simulink model "Airship_nonlinear_dynamics_simulink"  (R2024b)
settings: Solver=ode15s  StartTime=0.0  StopTime=1000  FixedStep=0.01  MaxStep=0.01  RelTol=1e-5  AbsTol=1e-8
InitFcn:
  | Init
values from neighbouring files (symbols this model uses):
  c = 0.465    [Init.m]    (also in Nonlinear_dynamics.m = 7; init_Skyship.m = 7)
  cf = 0.1395    [Init.m]    (also in Nonlinear_dynamics.m = 3; init_Skyship.m = 3)
  CL_alpha = 5.7    [Init.m]    (also in Nonlinear_dynamics.m; init_Skyship.m)
  D = 1.6    [Init.m]    (also in Nonlinear_dynamics.m = 14; init_Skyship.m = 14)
  delta = deg2rad(10)    [Nonlinear_dynamics.m]    (also in init_Skyship.m = -15)
  delta_e = 0    [Init.m]
  delta_r = 0    [Init.m]
  etaTDF = 1    [Init.m]    (also in Nonlinear_dynamics.m = 0.6; init_Skyship.m = 0.6)
  etaTP = 0.6    [Init.m]    (also in Nonlinear_dynamics.m; init_Skyship.m)
  fProp1 = 0    [Init.m]
  fProp2 = 0    [Init.m]
  fProp_max = 20    [Init.m]
  fTDF = 4000    [Nonlinear_dynamics.m]    (also in init_Skyship.m = 0)
  fTTP = 0    [Init.m]    (also in Nonlinear_dynamics.m = 2000; init_Skyship.m)
  FVN = [5, 5, 5]    [Init.m]    (also in Nonlinear_dynamics.m = 0; init_Skyship.m = 10)
  g = 9.81    [Init.m]    (also in Nonlinear_dynamics.m; init_Skyship.m)
  I33 = eye(3)    [Init.m]    (also in Nonlinear_dynamics.m; init_Skyship.m)
  Ixx = 1.7972    [Init.m]    (also in Nonlinear_dynamics.m = 200658; init_Skyship.m = 200658)
  Ixy = 0    [Init.m]    (also in Nonlinear_dynamics.m; init_Skyship.m)
  Ixz = 0    [Init.m]    (also in Nonlinear_dynamics.m; init_Skyship.m)
  Iyy = 4.9584    [Init.m]    (also in Nonlinear_dynamics.m = 850900; init_Skyship.m = 850900)
  Iyz = 0    [Init.m]    (also in Nonlinear_dynamics.m; init_Skyship.m)
  Izz = 7.9854    [Init.m]    (also in Nonlinear_dynamics.m = 649699; init_Skyship.m = 649699)
  k1 = keta(1)    [Init.m]    (also in Nonlinear_dynamics.m; init_Skyship.m = 0.08; ketaparameters.m = 0)
  k2 = keta(2)    [Init.m]    (also in Nonlinear_dynamics.m; init_Skyship.m = 0.89; ketaparameters.m = 0)
  k_dash = keta(3)    [Init.m]    (also in Nonlinear_dynamics.m; init_Skyship.m = 0.5; ketaparameters.m = 0)
  L = 4.7    [Init.m]    (also in Nonlinear_dynamics.m = zeros(1,4); init_Skyship.m = 52)
  m = 7.31    [Init.m]    (also in Nonlinear_dynamics.m = 5942; init_Skyship.m = 5942; velocity_tf_script.m; velocity_tf_script_v2.m)
  MAF = zeros(6,6)    [Init.m]    (also in Nonlinear_dynamics.m; init_Skyship.m)
  MVN = [0.2, 10, 5]    [Init.m]    (also in Nonlinear_dynamics.m = 0; init_Skyship.m = 0.001)
  p0 = 0    [Init.m]    (also in init_Skyship.m)
  phi0 = 0    [Init.m]    (also in init_Skyship.m)
  Prop1_alpha = 0    [Init.m]
  Prop2_alpha = 0    [Init.m]
  psi0 = 0    [Init.m]    (also in init_Skyship.m)
  q0 = 0    [Init.m]    (also in init_Skyship.m)
  r0 = 0    [Init.m]    (also in init_Skyship.m)
  rGxm = [XG-XB 0 ZG-ZB]'    [Init.m]    (also in Nonlinear_dynamics.m; init_Skyship.m)
  rho_0 = 1.225    [Init.m]    (also in Nonlinear_dynamics.m; init_Skyship.m)
  rho_he = 0.175    [Init.m]
  rTDF1 = [0 0.5 0]'    [Init.m]    (also in Nonlinear_dynamics.m = [3.5 7.87 21]'; init_Skyship.m = [3.5 7.87 21]')
  rTDF2 = [0 -0.5 0]'    [Init.m]    (also in Nonlinear_dynamics.m = [3.5 -7.87 21]'; init_Skyship.m = [3.5 -7.87 21]')
  rTTP = [0 0 0]'    [Init.m]    (also in Nonlinear_dynamics.m = [0 0 20.1]'; init_Skyship.m = [0 0 20.1]')
  Sf = 0.18135    [Init.m]    (also in Nonlinear_dynamics.m = 65; init_Skyship.m = 65)
  t_s = 0.005    [Init.m]
  theta0 = 1    [Init.m]    (also in init_Skyship.m = 0)
  u0 = 0.0    (= 0)    [Init.m]    (also in init_Skyship.m; velocity_tf_script.m = 4; velocity_tf_script_v2.m = 4)
  v0 = 0.0    (= 0)    [Init.m]    (also in init_Skyship.m)
  VB = 5.97    [Init.m]    (also in Nonlinear_dynamics.m = 5153; init_Skyship.m = 4911)
  w0 = 0.0    (= 0)    [Init.m]    (also in init_Skyship.m)
  xE0 = 0    [Init.m]    (also in init_Skyship.m)
  yE0 = 0    [Init.m]    (also in init_Skyship.m)
  zE0 = -h    (= -3.7495)    [Init.m]    (also in init_Skyship.m = -100)
undefined symbols (not defined in the file or in its folder): Sim3dSensor
libraries: slpidlib x13, simulink_extras x4, sim3dcameralib x1, sim3dlib x1, uavsim3dlib x1
(part 2 of 4)

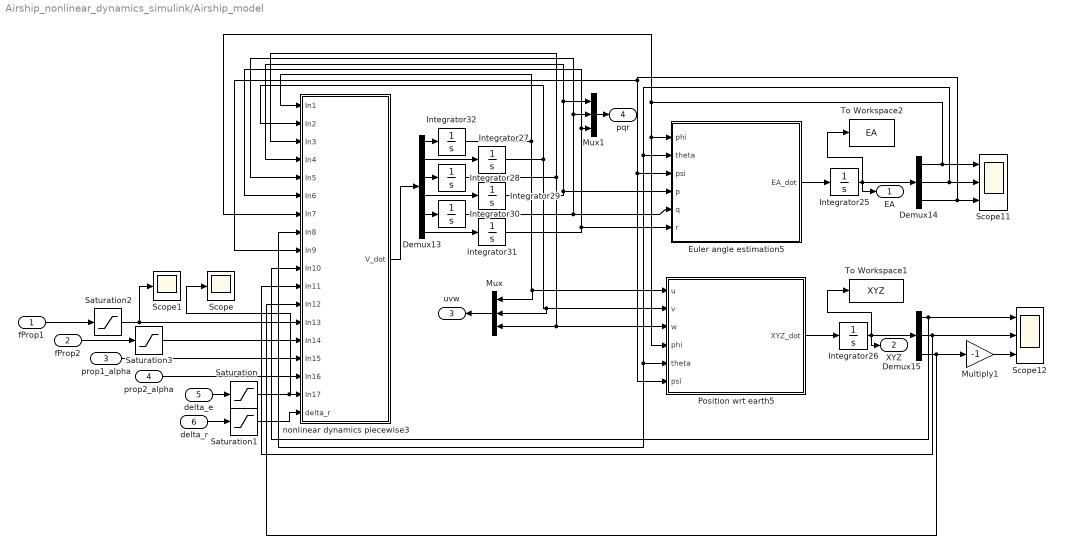
== system Airship_nonlinear_dynamics_simulink/Airship_model ==
  fProp1 : Inport
  fProp2 : Inport  Port=2
  prop1_alpha : Inport  Port=3
  prop2_alpha : Inport  Port=4
  delta_e : Inport  Port=5
  delta_r : Inport  Port=6
  Demux13 : Demux  Outputs=6
  Demux14 : Demux  Outputs=3
  Demux15 : Demux  Outputs=3
  Euler angle estimation5 : MATLAB Function  TreatAsAtomicUnit=on
  Integrator25 : Integrator  InitialCondition=[phi0 theta0 psi0]
  Integrator26 : Integrator  InitialCondition=[xE0 yE0 zE0]
  Integrator27 : Integrator  InitialCondition=v0
  Integrator28 : Integrator  InitialCondition=w0
  Integrator29 : Integrator  InitialCondition=p0
  Integrator30 : Integrator  InitialCondition=q0
  Integrator31 : Integrator  InitialCondition=r0
  Integrator32 : Integrator  InitialCondition=u0
  Multiply1 : Gain  Gain=-1
  Mux : Mux  Inputs=3
  Mux1 : Mux  Inputs=3
  Position wrt earth5 : MATLAB Function  TreatAsAtomicUnit=on
  Saturation : Saturate  UpperLimit=60  LowerLimit=-60
  Saturation1 : Saturate  UpperLimit=60  LowerLimit=-60
  Saturation2 : Saturate  UpperLimit=fProp_max  LowerLimit=-fProp_max
  Saturation3 : Saturate  UpperLimit=fProp_max  LowerLimit=-fProp_max
  Scope : Scope
  Scope1 : Scope
  Scope11 : Scope  NumInputPorts=3
  Scope12 : Scope  NumInputPorts=3
  To Workspace1 : ToWorkspace  VariableName=XYZ  SaveFormat=Timeseries  SampleTime=t_s
  To Workspace2 : ToWorkspace  VariableName=EA  SaveFormat=Timeseries  SampleTime=t_s
  nonlinear dynamics piecewise3 : Subsystem
  EA : Outport
  XYZ : Outport  Port=2
  uvw : Outport  Port=3
  pqr : Outport  Port=4
  wires:
  Demux13/5 -> Integrator30/1
  Integrator27/1 -> nonlinear dynamics piecewise3/2(In2), Position wrt earth5/2(v), Mux/2
  Demux14/2 -> Scope11/2, nonlinear dynamics piecewise3/8(In8), Position wrt earth5/5(theta), Euler angle estimation5/2(theta)
  Demux14/1 -> Scope11/1, nonlinear dynamics piecewise3/7(In7), Position wrt earth5/4(phi), Euler angle estimation5/1(phi)
  Demux13/6 -> Integrator31/1
  Integrator31/1 -> nonlinear dynamics piecewise3/6(In6), Mux1/3, Euler angle estimation5/6(r)
  delta_e/1 -> Saturation/1
  Position wrt earth5/1(XYZ_dot) -> Integrator26/1
  Demux14/3 -> Scope11/3, Euler angle estimation5/3(psi), Position wrt earth5/6(psi), nonlinear dynamics piecewise3/9(In9)
  Integrator28/1 -> nonlinear dynamics piecewise3/3(In3), Position wrt earth5/3(w), Mux/3
  Demux13/4 -> Integrator29/1
  Euler angle estimation5/1(EA_dot) -> Integrator25/1
  Integrator26/1 -> To Workspace1/1, XYZ/1, Demux15/1
  nonlinear dynamics piecewise3/1(V_dot) -> Demux13/1
  Integrator32/1 -> nonlinear dynamics piecewise3/1(In1), Position wrt earth5/1(u), Mux/1
  Demux15/1 -> Scope12/1, nonlinear dynamics piecewise3/10(In10)
  Multiply1/1 -> Scope12/3
  Demux13/1 -> Integrator32/1
  Demux13/2 -> Integrator27/1
  Demux13/3 -> Integrator28/1
  Integrator25/1 -> Demux14/1, EA/1, To Workspace2/1
  Demux15/2 -> nonlinear dynamics piecewise3/11(In11), Scope12/2
  Demux15/3 -> nonlinear dynamics piecewise3/12(In12), Multiply1/1
  fProp1/1 -> Saturation2/1
  prop1_alpha/1 -> nonlinear dynamics piecewise3/15(In15)
  fProp2/1 -> Saturation3/1
  prop2_alpha/1 -> nonlinear dynamics piecewise3/16(In16)
  Mux/1 -> uvw/1
  Integrator29/1 -> Euler angle estimation5/4(p), nonlinear dynamics piecewise3/4(In4), Mux1/1
  Integrator30/1 -> nonlinear dynamics piecewise3/5(In5), Mux1/2, Euler angle estimation5/5(q)
  Mux1/1 -> pqr/1
  delta_r/1 -> Saturation1/1
  Saturation/1 -> Scope/1, nonlinear dynamics piecewise3/17(In17)
  Saturation1/1 -> nonlinear dynamics piecewise3/18(delta_r)
  Saturation2/1 -> Scope1/1, nonlinear dynamics piecewise3/13(In13)
  Saturation3/1 -> nonlinear dynamics piecewise3/14(In14)

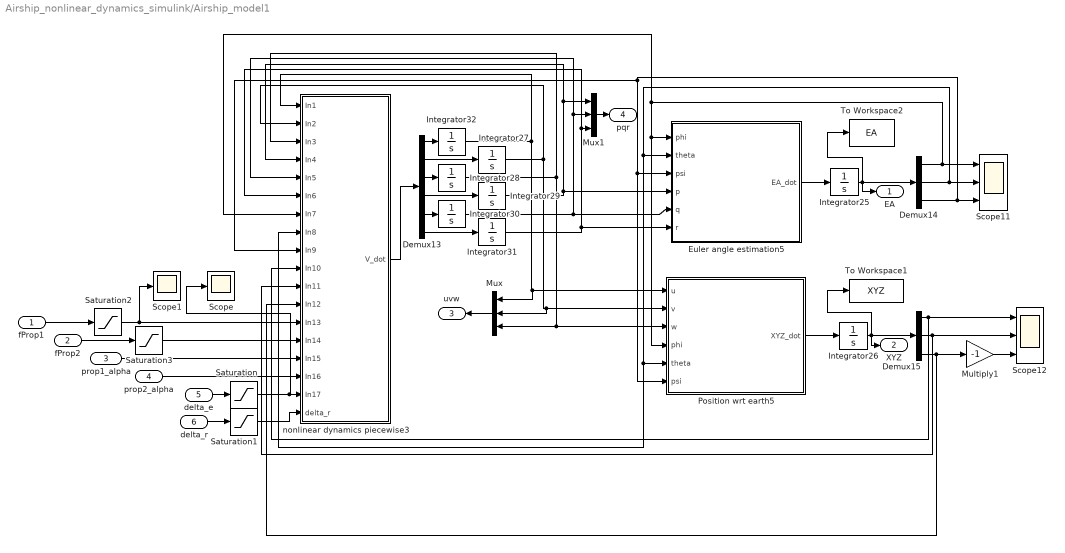
== system Airship_nonlinear_dynamics_simulink/Airship_model1 ==
  fProp1 : Inport
  fProp2 : Inport  Port=2
  prop1_alpha : Inport  Port=3
  prop2_alpha : Inport  Port=4
  delta_e : Inport  Port=5
  delta_r : Inport  Port=6
  Demux13 : Demux  Outputs=6
  Demux14 : Demux  Outputs=3
  Demux15 : Demux  Outputs=3
  Euler angle estimation5 : MATLAB Function  TreatAsAtomicUnit=on
  Integrator25 : Integrator  InitialCondition=[phi0 theta0 psi0]
  Integrator26 : Integrator  InitialCondition=[xE0 yE0 zE0]
  Integrator27 : Integrator  InitialCondition=v0
  Integrator28 : Integrator  InitialCondition=w0
  Integrator29 : Integrator  InitialCondition=p0
  Integrator30 : Integrator  InitialCondition=q0
  Integrator31 : Integrator  InitialCondition=r0
  Integrator32 : Integrator  InitialCondition=u0
  Multiply1 : Gain  Gain=-1
  Mux : Mux  Inputs=3
  Mux1 : Mux  Inputs=3
  Position wrt earth5 : MATLAB Function  TreatAsAtomicUnit=on
  Saturation : Saturate  UpperLimit=60  LowerLimit=-60
  Saturation1 : Saturate  UpperLimit=60  LowerLimit=-60
  Saturation2 : Saturate  UpperLimit=fProp_max  LowerLimit=-fProp_max
  Saturation3 : Saturate  UpperLimit=fProp_max  LowerLimit=-fProp_max
  Scope : Scope
  Scope1 : Scope
  Scope11 : Scope  NumInputPorts=3
  Scope12 : Scope  NumInputPorts=3
  To Workspace1 : ToWorkspace  VariableName=XYZ  SaveFormat=Timeseries  SampleTime=t_s
  To Workspace2 : ToWorkspace  VariableName=EA  SaveFormat=Timeseries  SampleTime=t_s
  nonlinear dynamics piecewise3 : Subsystem
  EA : Outport
  XYZ : Outport  Port=2
  uvw : Outport  Port=3
  pqr : Outport  Port=4
  wires:
  Demux13/5 -> Integrator30/1
  Integrator27/1 -> nonlinear dynamics piecewise3/2(In2), Position wrt earth5/2(v), Mux/2
  Demux14/2 -> Scope11/2, nonlinear dynamics piecewise3/8(In8), Position wrt earth5/5(theta), Euler angle estimation5/2(theta)
  Demux14/1 -> Scope11/1, nonlinear dynamics piecewise3/7(In7), Position wrt earth5/4(phi), Euler angle estimation5/1(phi)
  Demux13/6 -> Integrator31/1
  Integrator31/1 -> nonlinear dynamics piecewise3/6(In6), Mux1/3, Euler angle estimation5/6(r)
  delta_e/1 -> Saturation/1
  Position wrt earth5/1(XYZ_dot) -> Integrator26/1
  Demux14/3 -> Scope11/3, Euler angle estimation5/3(psi), Position wrt earth5/6(psi), nonlinear dynamics piecewise3/9(In9)
  Integrator28/1 -> nonlinear dynamics piecewise3/3(In3), Position wrt earth5/3(w), Mux/3
  Demux13/4 -> Integrator29/1
  Euler angle estimation5/1(EA_dot) -> Integrator25/1
  Integrator26/1 -> To Workspace1/1, XYZ/1, Demux15/1
  nonlinear dynamics piecewise3/1(V_dot) -> Demux13/1
  Integrator32/1 -> nonlinear dynamics piecewise3/1(In1), Position wrt earth5/1(u), Mux/1
  Demux15/1 -> Scope12/1, nonlinear dynamics piecewise3/10(In10)
  Multiply1/1 -> Scope12/3
  Demux13/1 -> Integrator32/1
  Demux13/2 -> Integrator27/1
  Demux13/3 -> Integrator28/1
  Integrator25/1 -> Demux14/1, EA/1, To Workspace2/1
  Demux15/2 -> nonlinear dynamics piecewise3/11(In11), Scope12/2
  Demux15/3 -> nonlinear dynamics piecewise3/12(In12), Multiply1/1
  fProp1/1 -> Saturation2/1
  prop1_alpha/1 -> nonlinear dynamics piecewise3/15(In15)
  fProp2/1 -> Saturation3/1
  prop2_alpha/1 -> nonlinear dynamics piecewise3/16(In16)
  Mux/1 -> uvw/1
  Integrator29/1 -> Euler angle estimation5/4(p), nonlinear dynamics piecewise3/4(In4), Mux1/1
  Integrator30/1 -> nonlinear dynamics piecewise3/5(In5), Mux1/2, Euler angle estimation5/5(q)
  Mux1/1 -> pqr/1
  delta_r/1 -> Saturation1/1
  Saturation/1 -> Scope/1, nonlinear dynamics piecewise3/17(In17)
  Saturation1/1 -> nonlinear dynamics piecewise3/18(delta_r)
  Saturation2/1 -> Scope1/1, nonlinear dynamics piecewise3/13(In13)
  Saturation3/1 -> nonlinear dynamics piecewise3/14(In14)

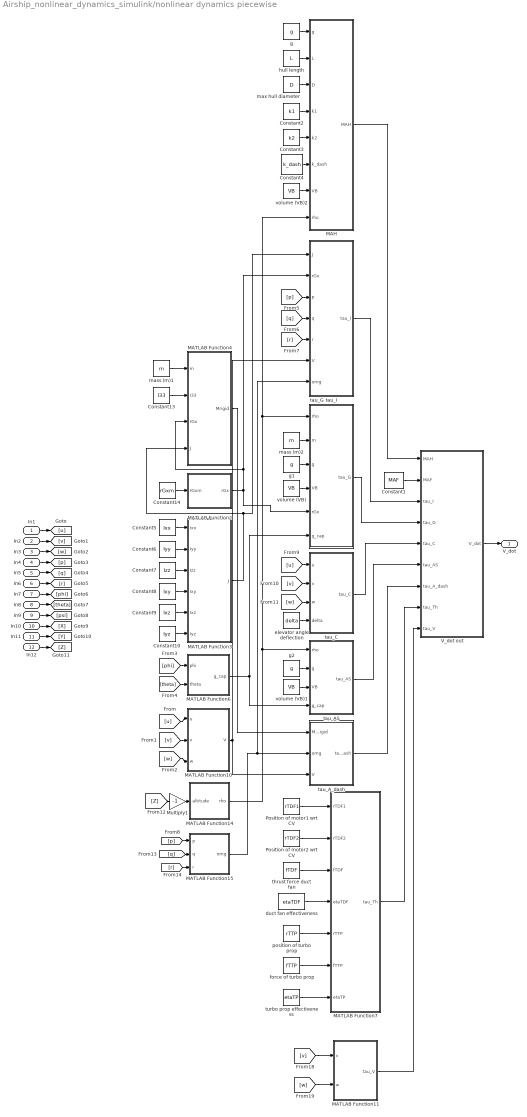
== system Airship_nonlinear_dynamics_simulink/nonlinear dynamics piecewise ==
  In1 : Inport
  In2 : Inport  Port=2
  In3 : Inport  Port=3
  In4 : Inport  Port=4
  In5 : Inport  Port=5
  In6 : Inport  Port=6
  In7 : Inport  Port=7
  In8 : Inport  Port=8
  In9 : Inport  Port=9
  In10 : Inport  Port=10
  In11 : Inport  Port=11
  In12 : Inport  Port=12
  Constant1 : Constant  Value=MAF
  Constant10 : Constant  Value=Iyz
  Constant13 : Constant  Value=I33
  Constant14 : Constant  Value=rGxm
  Constant2 : Constant  Value=k1
  Constant3 : Constant  Value=k2
  Constant4 : Constant  Value=k_dash
  Constant5 : Constant  Value=Ixx
  Constant6 : Constant  Value=Iyy
  Constant7 : Constant  Value=Izz
  Constant8 : Constant  Value=Ixy
  Constant9 : Constant  Value=Ixz
  MAH : MATLAB Function  TreatAsAtomicUnit=on
  MATLAB Function10 : MATLAB Function  TreatAsAtomicUnit=on
  MATLAB Function11 : MATLAB Function  TreatAsAtomicUnit=on
  MATLAB Function14 : MATLAB Function  TreatAsAtomicUnit=on
  MATLAB Function15 : MATLAB Function  TreatAsAtomicUnit=on
  MATLAB Function2 : MATLAB Function  TreatAsAtomicUnit=on
  MATLAB Function3 : MATLAB Function  TreatAsAtomicUnit=on
  MATLAB Function4 : MATLAB Function  TreatAsAtomicUnit=on
  MATLAB Function6 : MATLAB Function  TreatAsAtomicUnit=on
  MATLAB Function7 : MATLAB Function  TreatAsAtomicUnit=on
  Multiply1 : Gain  Gain=-1
  Position of motor1 wrt CV : Constant  Value=rTDF1
  Position of motor2 wrt CV : Constant  Value=rTDF2
  V_dot out : MATLAB Function  TreatAsAtomicUnit=on
  duct fan effectiveness : Constant  Value=etaTDF
  elevator angle deflection : Constant  Value=delta
  force of turbo prop : Constant  Value=fTTP
  g : Constant  Value=g
  g1 : Constant  Value=g
  g2 : Constant  Value=g
  hull length : Constant  Value=L
  mass (m)1 : Constant  Value=m
  mass (m)2 : Constant  Value=m
  max hull diameter : Constant  Value=D
  position of turbo prop : Constant  Value=rTTP
  tau_AS : MATLAB Function  TreatAsAtomicUnit=on
  tau_A_dash : MATLAB Function  TreatAsAtomicUnit=on
  tau_C : MATLAB Function  TreatAsAtomicUnit=on
  tau_G : MATLAB Function  TreatAsAtomicUnit=on
  tau_I : MATLAB Function  TreatAsAtomicUnit=on
  thrust force duct fan : Constant  Value=fTDF
  turbo prop effectiveness : Constant  Value=etaTP
  volume (VB) : Constant  Value=VB
  volume (VB)1 : Constant  Value=VB
  volume (VB)2 : Constant  Value=VB
  V_dot : Outport
  wires:
  V_dot out/1(V_dot) -> V_dot/1
  Constant1/1 -> V_dot out/2(MAF)
  In1/1 -> [u]
  In2/1 -> [v]
  In3/1 -> [w]
  In4/1 -> [p]
  In5/1 -> [q]
  In6/1 -> [r]
  In7/1 -> [phi]
  In8/1 -> [theta]
  In9/1 -> [psi]
  In10/1 -> [X]
  In11/1 -> [Y]
  In12/1 -> [Z]
  mass (m)1/1 -> MATLAB Function4/1(m)
  mass (m)2/1 -> tau_G/2(m)
  Constant13/1 -> MATLAB Function4/2(I33)
  Constant14/1 -> MATLAB Function2/1(rGxm)
  MATLAB Function2/1(rGx) -> tau_G/5(rGx), MATLAB Function4/3(rGx), tau_I/2(rGx)
  MATLAB Function3/1(J) -> MATLAB Function4/4(J), tau_I/1(J)
  Constant6/1 -> MATLAB Function3/2(Iyy)
  Constant5/1 -> MATLAB Function3/1(Ixx)
  Constant7/1 -> MATLAB Function3/3(Izz)
  Constant8/1 -> MATLAB Function3/4(Ixy)
  Constant9/1 -> MATLAB Function3/5(Ixz)
  Constant10/1 -> MATLAB Function3/6(Iyz)
  [u] -> MATLAB Function10/1(u)
  [v] -> MATLAB Function10/2(v)
  [w] -> MATLAB Function10/3(w)
  [phi] -> MATLAB Function6/1(phi)
  [theta] -> MATLAB Function6/2(theta)
  g/1 -> MAH/1(g)
  hull length/1 -> MAH/2(L)
  max hull diameter/1 -> MAH/3(D)
  Constant2/1 -> MAH/4(k1)
  Constant3/1 -> MAH/5(k2)
  [p] -> tau_I/3(p)
  [q] -> tau_I/4(q)
  [r] -> tau_I/5(r)
  MATLAB Function10/1(V) -> tau_A_dash/3(V), tau_I/6(V)
  MATLAB Function14/1(rho) -> tau_AS/1(rho), MAH/8(rho), tau_G/1(rho)
  g1/1 -> tau_G/3(g)
  volume (VB)/1 -> tau_G/4(VB)
  MATLAB Function6/1(g_cap) -> tau_AS/4(g_cap), tau_G/6(g_cap)
  [u] -> tau_C/1(u)
  [v] -> tau_C/2(v)
  [w] -> tau_C/3(w)
  elevator angle deflection/1 -> tau_C/4(delta)
  [Z] -> Multiply1/1
  Multiply1/1 -> MATLAB Function14/1(altitude)
  g2/1 -> tau_AS/2(g)
  volume (VB)1/1 -> tau_AS/3(VB)
  MATLAB Function4/1(Mrigid) -> tau_A_dash/1(MA_rigid)
  [p] -> MATLAB Function15/1(p)
  [q] -> MATLAB Function15/2(q)
  [r] -> MATLAB Function15/3(r)
  MATLAB Function15/1(omg) -> tau_A_dash/2(omg), tau_I/7(omg)
  Position of motor1 wrt CV/1 -> MATLAB Function7/1(rTDF1)
  Position of motor2 wrt CV/1 -> MATLAB Function7/2(rTDF2)
  thrust force duct fan/1 -> MATLAB Function7/3(fTDF)
  duct fan effectiveness/1 -> MATLAB Function7/4(etaTDF)
  position of turbo prop/1 -> MATLAB Function7/5(rTTP)
  force of turbo prop/1 -> MATLAB Function7/6(fTTP)
  turbo prop effectiveness/1 -> MATLAB Function7/7(etaTP)
  [v] -> MATLAB Function11/1(v)
  [w] -> MATLAB Function11/2(w)
  Constant4/1 -> MAH/6(k_dash)
  MAH/1(MAH) -> V_dot out/1(MAH)
  tau_I/1(tau_I) -> V_dot out/3(tau_I)
  tau_G/1(tau_G) -> V_dot out/4(tau_G)
  tau_C/1(tau_C) -> V_dot out/5(tau_C)
  tau_AS/1(tau_AS) -> V_dot out/6(tau_AS)
  tau_A_dash/1(tau_A_dash) -> V_dot out/7(tau_A_dash)
  MATLAB Function7/1(tau_Th) -> V_dot out/8(tau_Th)
  MATLAB Function11/1(tau_V) -> V_dot out/9(tau_V)
  volume (VB)2/1 -> MAH/7(VB)

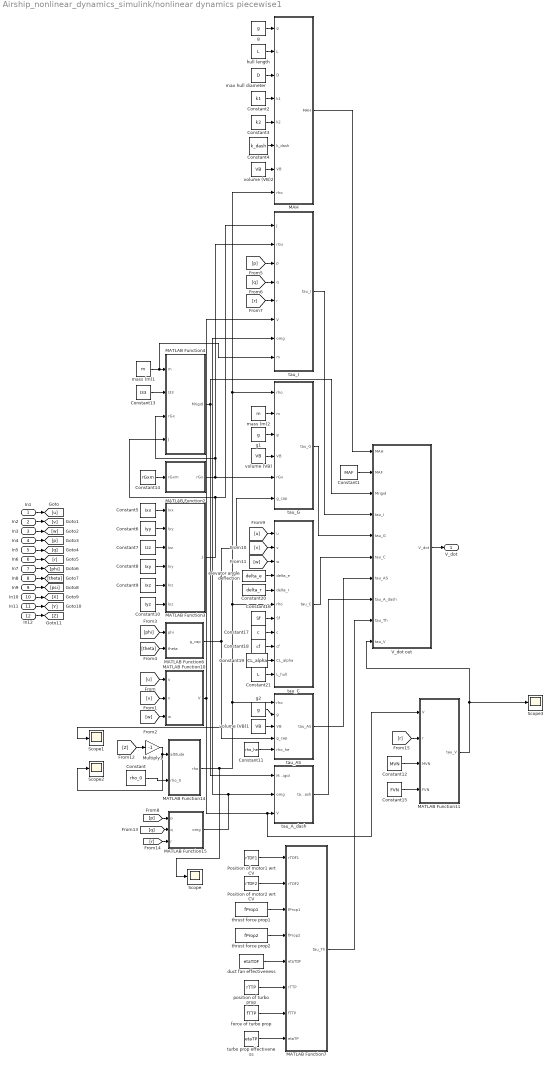
== system Airship_nonlinear_dynamics_simulink/nonlinear dynamics piecewise1 ==
  In1 : Inport
  In2 : Inport  Port=2
  In3 : Inport  Port=3
  In4 : Inport  Port=4
  In5 : Inport  Port=5
  In6 : Inport  Port=6
  In7 : Inport  Port=7
  In8 : Inport  Port=8
  In9 : Inport  Port=9
  In10 : Inport  Port=10
  In11 : Inport  Port=11
  In12 : Inport  Port=12
  Constant : Constant  Value=rho_0
  Constant1 : Constant  Value=MAF
  Constant10 : Constant  Value=Iyz
  Constant11 : Constant  Value=rho_he
  Constant12 : Constant  Value=MVN
  Constant13 : Constant  Value=I33
  Constant14 : Constant  Value=rGxm
  Constant15 : Constant  Value=FVN
  Constant16 : Constant  Value=Sf
  Constant17 : Constant  Value=c
  Constant18 : Constant  Value=cf
  Constant19 : Constant  Value=CL_alpha
  Constant2 : Constant  Value=k1
  Constant20 : Constant  Value=delta_r
  Constant21 : Constant  Value=L
  Constant3 : Constant  Value=k2
  Constant4 : Constant  Value=k_dash
  Constant5 : Constant  Value=Ixx
  Constant6 : Constant  Value=Iyy
  Constant7 : Constant  Value=Izz
  Constant8 : Constant  Value=Ixy
  Constant9 : Constant  Value=Ixz
  MAH : MATLAB Function  TreatAsAtomicUnit=on
  MATLAB Function10 : MATLAB Function  TreatAsAtomicUnit=on
  MATLAB Function11 : MATLAB Function  TreatAsAtomicUnit=on
  MATLAB Function14 : MATLAB Function  TreatAsAtomicUnit=on
  MATLAB Function15 : MATLAB Function  TreatAsAtomicUnit=on
  MATLAB Function2 : MATLAB Function  TreatAsAtomicUnit=on
  MATLAB Function3 : MATLAB Function  TreatAsAtomicUnit=on
  MATLAB Function4 : MATLAB Function  TreatAsAtomicUnit=on
  MATLAB Function6 : MATLAB Function  TreatAsAtomicUnit=on
  MATLAB Function7 : MATLAB Function  TreatAsAtomicUnit=on
  Multiply1 : Gain  Gain=-1
  Position of motor1 wrt CV : Constant  Value=rTDF1
  Position of motor2 wrt CV : Constant  Value=rTDF2
  Scope{,1..3} (4 alike) : Scope
  V_dot out : MATLAB Function  TreatAsAtomicUnit=on
  duct fan effectiveness : Constant  Value=etaTDF
  elevator angle deflection : Constant  Value=delta_e
  force of turbo prop : Constant  Value=fTTP
  g : Constant  Value=g
  g1 : Constant  Value=g
  g2 : Constant  Value=g
  hull length : Constant  Value=L
  mass (m)1 : Constant  Value=m
  mass (m)2 : Constant  Value=m
  max hull diameter : Constant  Value=D
  position of turbo prop : Constant  Value=rTTP
  tau_AS : MATLAB Function  TreatAsAtomicUnit=on
  tau_A_dash : MATLAB Function  TreatAsAtomicUnit=on
  tau_C : MATLAB Function  TreatAsAtomicUnit=on
  tau_G : MATLAB Function  TreatAsAtomicUnit=on
  tau_I : MATLAB Function  TreatAsAtomicUnit=on
  thrust force prop1 : Constant  Value=fProp1
  thrust force prop2 : Constant  Value=fProp2
  turbo prop effectiveness : Constant  Value=etaTP
  volume (VB) : Constant  Value=VB
  volume (VB)1 : Constant  Value=VB
  volume (VB)2 : Constant  Value=VB
  V_dot : Outport
  wires:
  V_dot out/1(V_dot) -> V_dot/1
  Constant1/1 -> V_dot out/2(MAF)
  In1/1 -> [u]
  In2/1 -> [v]
  In3/1 -> [w]
  In4/1 -> [p]
  In5/1 -> [q]
  In6/1 -> [r]
  In7/1 -> [phi]
  In8/1 -> [theta]
  In9/1 -> [psi]
  In10/1 -> [X]
  In11/1 -> [Y]
  In12/1 -> [Z]
  mass (m)1/1 -> tau_I/8(m), MATLAB Function4/1(m)
  mass (m)2/1 -> tau_G/2(m)
  Constant13/1 -> MATLAB Function4/2(I33)
  Constant14/1 -> MATLAB Function2/1(rGxm)
  MATLAB Function2/1(rGx) -> tau_G/5(rGx), MATLAB Function4/3(rGx), tau_I/2(rGx)
  MATLAB Function3/1(J) -> MATLAB Function4/4(J), tau_I/1(J)
  Constant6/1 -> MATLAB Function3/2(Iyy)
  Constant5/1 -> MATLAB Function3/1(Ixx)
  Constant7/1 -> MATLAB Function3/3(Izz)
  Constant8/1 -> MATLAB Function3/4(Ixy)
  Constant9/1 -> MATLAB Function3/5(Ixz)
  Constant10/1 -> MATLAB Function3/6(Iyz)
  [u] -> MATLAB Function10/1(u)
  [v] -> MATLAB Function10/2(v)
  [w] -> MATLAB Function10/3(w)
  [phi] -> MATLAB Function6/1(phi)
  [theta] -> MATLAB Function6/2(theta)
  g/1 -> MAH/1(g)
  hull length/1 -> MAH/2(L)
  max hull diameter/1 -> MAH/3(D)
  Constant2/1 -> MAH/4(k1)
  Constant3/1 -> MAH/5(k2)
  [p] -> tau_I/3(p)
  [q] -> tau_I/4(q)
  [r] -> tau_I/5(r)
  MATLAB Function14/1(rho) -> Scope1/1, MAH/8(rho), tau_G/1(rho), tau_C/6(rho), tau_AS/1(rho), Scope/1
  g1/1 -> tau_G/3(g)
  volume (VB)/1 -> tau_G/4(VB)
  MATLAB Function6/1(g_cap) -> tau_AS/4(g_cap), tau_G/6(g_cap)
  [u] -> tau_C/1(u)
  [v] -> tau_C/2(v)
  [w] -> tau_C/3(w)
  elevator angle deflection/1 -> tau_C/4(delta_e)
  [Z] -> Multiply1/1
  Multiply1/1 -> Scope2/1, MATLAB Function14/1(altitude)
  g2/1 -> tau_AS/2(g)
  volume (VB)1/1 -> tau_AS/3(VB)
  MATLAB Function4/1(Mrigid) -> tau_A_dash/1(MA_rigid), V_dot out/3(Mrigid)
  [p] -> MATLAB Function15/1(p)
  [q] -> MATLAB Function15/2(q)
  [r] -> MATLAB Function15/3(r)
  MATLAB Function15/1(omg) -> tau_I/7(omg), tau_A_dash/2(omg)
  Position of motor1 wrt CV/1 -> MATLAB Function7/1(rTDF1)
  Position of motor2 wrt CV/1 -> MATLAB Function7/2(rTDF2)
  thrust force prop1/1 -> MATLAB Function7/3(fProp1)
  duct fan effectiveness/1 -> MATLAB Function7/5(etaTDF)
  position of turbo prop/1 -> MATLAB Function7/6(rTTP)
  force of turbo prop/1 -> MATLAB Function7/7(fTTP)
  turbo prop effectiveness/1 -> MATLAB Function7/8(etaTP)
  MATLAB Function10/1(V) -> MATLAB Function11/1(V), tau_A_dash/3(V), tau_I/6(V)
  Constant4/1 -> MAH/6(k_dash)
  MAH/1(MAH) -> V_dot out/1(MAH)
  tau_I/1(tau_I) -> V_dot out/4(tau_I)
  tau_G/1(tau_G) -> V_dot out/5(tau_G)
  tau_AS/1(tau_AS) -> V_dot out/7(tau_AS)
  tau_A_dash/1(tau_A_dash) -> V_dot out/8(tau_A_dash)
  MATLAB Function7/1(tau_Th) -> V_dot out/9(tau_Th)
  MATLAB Function11/1(tau_V) -> Scope3/1, V_dot out/10(tau_V)
  volume (VB)2/1 -> MAH/7(VB)
  Constant/1 -> MATLAB Function14/2(rho_0)
  Constant16/1 -> tau_C/7(Sf)
  Constant17/1 -> tau_C/8(c)
  Constant18/1 -> tau_C/9(cf)
  Constant19/1 -> tau_C/10(CL_alpha)
  Constant11/1 -> tau_AS/5(rho_he)
  tau_C/1(tau_C) -> V_dot out/6(tau_C)
  Constant15/1 -> MATLAB Function11/4(FVN)
  Constant12/1 -> MATLAB Function11/3(MVN)
  Constant20/1 -> tau_C/5(delta_r)
  Constant21/1 -> tau_C/11(L_hull)
  [r] -> MATLAB Function11/2(r)
  thrust force prop2/1 -> MATLAB Function7/4(fProp2)

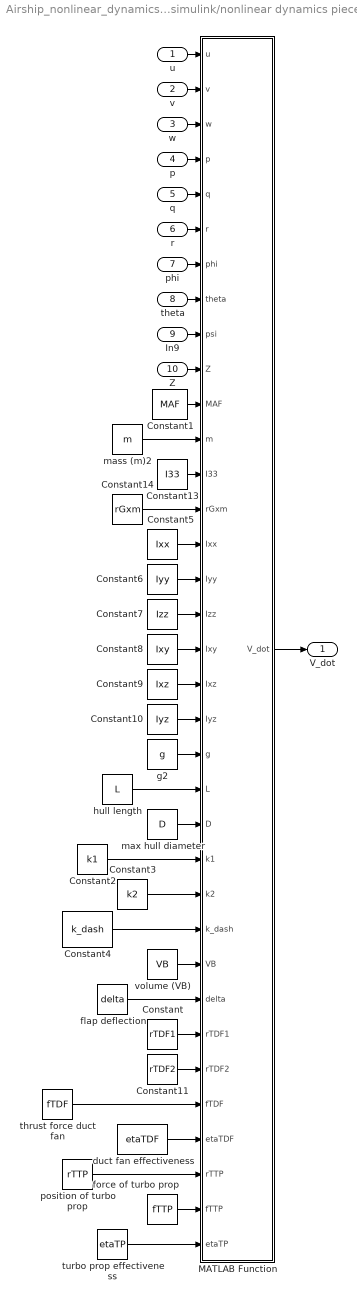
== system Airship_nonlinear_dynamics_simulink/nonlinear dynamics piecewise2 ==
  u : Inport
  v : Inport  Port=2
  w : Inport  Port=3
  p : Inport  Port=4
  q : Inport  Port=5
  r : Inport  Port=6
  phi : Inport  Port=7
  theta : Inport  Port=8
  In9 : Inport  Port=9
  Z : Inport  Port=10
  Constant : Constant  Value=rTDF1
  Constant1 : Constant  Value=MAF
  Constant10 : Constant  Value=Iyz
  Constant11 : Constant  Value=rTDF2
  Constant13 : Constant  Value=I33
  Constant14 : Constant  Value=rGxm
  Constant2 : Constant  Value=k1
  Constant3 : Constant  Value=k2
  Constant4 : Constant  Value=k_dash
  Constant5 : Constant  Value=Ixx
  Constant6 : Constant  Value=Iyy
  Constant7 : Constant  Value=Izz
  Constant8 : Constant  Value=Ixy
  Constant9 : Constant  Value=Ixz
  MATLAB Function : MATLAB Function  TreatAsAtomicUnit=on
  duct fan effectiveness : Constant  Value=etaTDF
  flap deflection : Constant  Value=delta
  force of turbo prop : Constant  Value=fTTP
  g2 : Constant  Value=g
  hull length : Constant  Value=L
  mass (m)2 : Constant  Value=m
  max hull diameter : Constant  Value=D
  position of turbo prop : Constant  Value=rTTP
  thrust force duct fan : Constant  Value=fTDF
  turbo prop effectiveness : Constant  Value=etaTP
  volume (VB) : Constant  Value=VB
  V_dot : Outport
  wires:
  MATLAB Function/1(V_dot) -> V_dot/1
  mass (m)2/1 -> MATLAB Function/12(m)
  Constant6/1 -> MATLAB Function/16(Iyy)
  Constant5/1 -> MATLAB Function/15(Ixx)
  Constant7/1 -> MATLAB Function/17(Izz)
  Constant8/1 -> MATLAB Function/18(Ixy)
  Constant9/1 -> MATLAB Function/19(Ixz)
  Constant10/1 -> MATLAB Function/20(Iyz)
  Constant4/1 -> MATLAB Function/26(k_dash)
  u/1 -> MATLAB Function/1(u)
  v/1 -> MATLAB Function/2(v)
  Constant1/1 -> MATLAB Function/11(MAF)
  Constant13/1 -> MATLAB Function/13(I33)
  g2/1 -> MATLAB Function/21(g)
  Constant14/1 -> MATLAB Function/14(rGxm)
  hull length/1 -> MATLAB Function/22(L)
  max hull diameter/1 -> MATLAB Function/23(D)
  Constant2/1 -> MATLAB Function/24(k1)
  Constant3/1 -> MATLAB Function/25(k2)
  volume (VB)/1 -> MATLAB Function/27(VB)
  flap deflection/1 -> MATLAB Function/28(delta)
  force of turbo prop/1 -> MATLAB Function/34(fTTP)
  position of turbo prop/1 -> MATLAB Function/33(rTTP)
  duct fan effectiveness/1 -> MATLAB Function/32(etaTDF)
  turbo prop effectiveness/1 -> MATLAB Function/35(etaTP)
  thrust force duct fan/1 -> MATLAB Function/31(fTDF)
  Constant/1 -> MATLAB Function/29(rTDF1)
  Constant11/1 -> MATLAB Function/30(rTDF2)
  In9/1 -> MATLAB Function/9(psi)
  w/1 -> MATLAB Function/3(w)
  p/1 -> MATLAB Function/4(p)
  q/1 -> MATLAB Function/5(q)
  r/1 -> MATLAB Function/6(r)
  phi/1 -> MATLAB Function/7(phi)
  theta/1 -> MATLAB Function/8(theta)
  Z/1 -> MATLAB Function/10(Z)

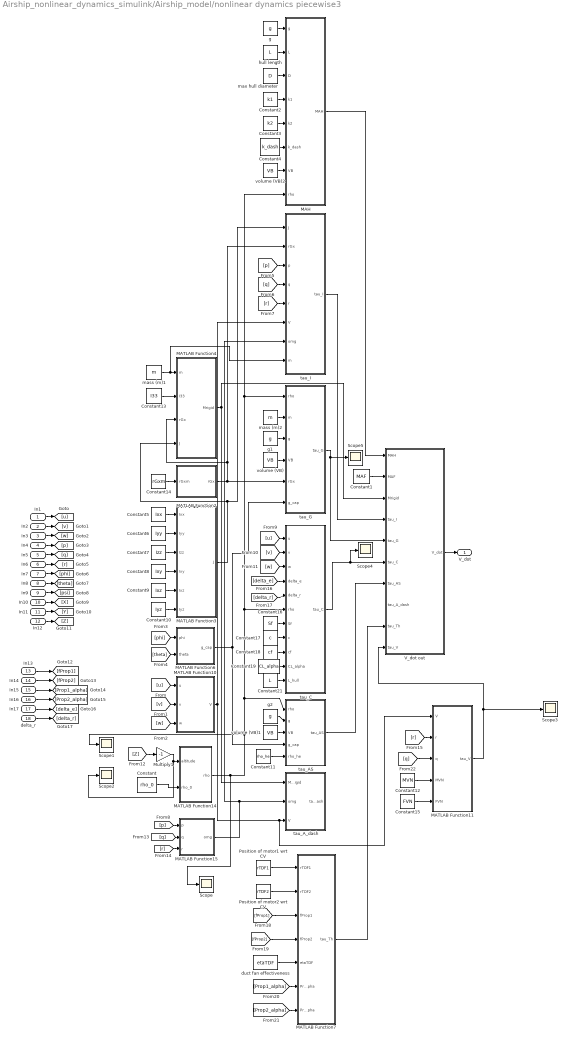
== system Airship_nonlinear_dynamics_simulink/Airship_model/nonlinear dynamics piecewise3 ==
  In1 : Inport
  In2 : Inport  Port=2
  In3 : Inport  Port=3
  In4 : Inport  Port=4
  In5 : Inport  Port=5
  In6 : Inport  Port=6
  In7 : Inport  Port=7
  In8 : Inport  Port=8
  In9 : Inport  Port=9
  In10 : Inport  Port=10
  In11 : Inport  Port=11
  In12 : Inport  Port=12
  In13 : Inport  Port=13
  In14 : Inport  Port=14
  In15 : Inport  Port=15
  In16 : Inport  Port=16
  In17 : Inport  Port=17
  delta_r : Inport  Port=18
  Constant : Constant  Value=rho_0
  Constant1 : Constant  Value=MAF
  Constant10 : Constant  Value=Iyz
  Constant11 : Constant  Value=rho_he
  Constant12 : Constant  Value=MVN
  Constant13 : Constant  Value=I33
  Constant14 : Constant  Value=rGxm
  Constant15 : Constant  Value=FVN
  Constant16 : Constant  Value=Sf
  Constant17 : Constant  Value=c
  Constant18 : Constant  Value=cf
  Constant19 : Constant  Value=CL_alpha
  Constant2 : Constant  Value=k1
  Constant21 : Constant  Value=L
  Constant3 : Constant  Value=k2
  Constant4 : Constant  Value=k_dash
  Constant5 : Constant  Value=Ixx
  Constant6 : Constant  Value=Iyy
  Constant7 : Constant  Value=Izz
  Constant8 : Constant  Value=Ixy
  Constant9 : Constant  Value=Ixz
  MAH : MATLAB Function  TreatAsAtomicUnit=on
  MATLAB Function10 : MATLAB Function  TreatAsAtomicUnit=on
  MATLAB Function11 : MATLAB Function  TreatAsAtomicUnit=on
  MATLAB Function14 : MATLAB Function  TreatAsAtomicUnit=on
  MATLAB Function15 : MATLAB Function  TreatAsAtomicUnit=on
  MATLAB Function2 : MATLAB Function  TreatAsAtomicUnit=on
  MATLAB Function3 : MATLAB Function  TreatAsAtomicUnit=on
  MATLAB Function4 : MATLAB Function  TreatAsAtomicUnit=on
  MATLAB Function6 : MATLAB Function  TreatAsAtomicUnit=on
  MATLAB Function7 : MATLAB Function  TreatAsAtomicUnit=on
  Multiply1 : Gain  Gain=-1
  Position of motor1 wrt CV : Constant  Value=rTDF1
  Position of motor2 wrt CV : Constant  Value=rTDF2
  Scope{,1..5} (6 alike) : Scope
  V_dot out : MATLAB Function  TreatAsAtomicUnit=on
  duct fan effectiveness : Constant  Value=etaTDF
  g : Constant  Value=g
  g1 : Constant  Value=g
  g2 : Constant  Value=g
  hull length : Constant  Value=L
  mass (m)1 : Constant  Value=m
  mass (m)2 : Constant  Value=m
  max hull diameter : Constant  Value=D
  tau_AS : MATLAB Function  TreatAsAtomicUnit=on
  tau_A_dash : MATLAB Function  TreatAsAtomicUnit=on
  tau_C : MATLAB Function  TreatAsAtomicUnit=on
  tau_G : MATLAB Function  TreatAsAtomicUnit=on
  tau_I : MATLAB Function  TreatAsAtomicUnit=on
  volume (VB) : Constant  Value=VB
  volume (VB)1 : Constant  Value=VB
  volume (VB)2 : Constant  Value=VB
  V_dot : Outport
  wires:
  V_dot out/1(V_dot) -> V_dot/1
  Constant1/1 -> V_dot out/2(MAF)
  In1/1 -> [u]
  In2/1 -> [v]
  In3/1 -> [w]
  In4/1 -> [p]
  In5/1 -> [q]
  In6/1 -> [r]
  In7/1 -> [phi]
  In8/1 -> [theta]
  In9/1 -> [psi]
  In10/1 -> [X]
  In11/1 -> [Y]
  In12/1 -> [Z]
  mass (m)1/1 -> tau_I/8(m), MATLAB Function4/1(m)
  mass (m)2/1 -> tau_G/2(m)
  Constant13/1 -> MATLAB Function4/2(I33)
  Constant14/1 -> MATLAB Function2/1(rGxm)
  MATLAB Function2/1(rGx) -> tau_G/5(rGx), MATLAB Function4/3(rGx), tau_I/2(rGx)
  MATLAB Function3/1(J) -> MATLAB Function4/4(J), tau_I/1(J)
  Constant6/1 -> MATLAB Function3/2(Iyy)
  Constant5/1 -> MATLAB Function3/1(Ixx)
  Constant7/1 -> MATLAB Function3/3(Izz)
  Constant8/1 -> MATLAB Function3/4(Ixy)
  Constant9/1 -> MATLAB Function3/5(Ixz)
  Constant10/1 -> MATLAB Function3/6(Iyz)
  [u] -> MATLAB Function10/1(u)
  [v] -> MATLAB Function10/2(v)
  [w] -> MATLAB Function10/3(w)
  [phi] -> MATLAB Function6/1(phi)
  [theta] -> MATLAB Function6/2(theta)
  g/1 -> MAH/1(g)
  hull length/1 -> MAH/2(L)
  max hull diameter/1 -> MAH/3(D)
  Constant2/1 -> MAH/4(k1)
  Constant3/1 -> MAH/5(k2)
  [p] -> tau_I/3(p)
  [q] -> tau_I/4(q)
  [r] -> tau_I/5(r)
  MATLAB Function14/1(rho) -> Scope1/1, MAH/8(rho), tau_G/1(rho), tau_C/6(rho), tau_AS/1(rho), Scope/1
  g1/1 -> tau_G/3(g)
  volume (VB)/1 -> tau_G/4(VB)
  MATLAB Function6/1(g_cap) -> tau_AS/4(g_cap), tau_G/6(g_cap)
  [u] -> tau_C/1(u)
  [v] -> tau_C/2(v)
  [w] -> tau_C/3(w)
  [delta_e] -> tau_C/4(delta_e)
  [Z] -> Multiply1/1
  Multiply1/1 -> Scope2/1, MATLAB Function14/1(altitude)
  g2/1 -> tau_AS/2(g)
  volume (VB)1/1 -> tau_AS/3(VB)
  MATLAB Function4/1(Mrigid) -> tau_A_dash/1(MA_rigid), V_dot out/3(Mrigid)
  [p] -> MATLAB Function15/1(p)
  [q] -> MATLAB Function15/2(q)
  [r] -> MATLAB Function15/3(r)
  MATLAB Function15/1(omg) -> tau_I/7(omg), tau_A_dash/2(omg)
  Position of motor1 wrt CV/1 -> MATLAB Function7/1(rTDF1)
  Position of motor2 wrt CV/1 -> MATLAB Function7/2(rTDF2)
  duct fan effectiveness/1 -> MATLAB Function7/5(etaTDF)
  [fProp1] -> MATLAB Function7/3(fProp1)
  MATLAB Function10/1(V) -> MATLAB Function11/1(V), tau_A_dash/3(V), tau_I/6(V)
  Constant4/1 -> MAH/6(k_dash)
  MAH/1(MAH) -> V_dot out/1(MAH)
  tau_I/1(tau_I) -> V_dot out/4(tau_I)
  tau_G/1(tau_G) -> Scope5/1, V_dot out/5(tau_G)
  tau_AS/1(tau_AS) -> V_dot out/7(tau_AS)
  MATLAB Function11/1(tau_V) -> V_dot out/10(tau_V), Scope3/1
  volume (VB)2/1 -> MAH/7(VB)
  Constant/1 -> MATLAB Function14/2(rho_0)
  Constant16/1 -> tau_C/7(Sf)
  Constant17/1 -> tau_C/8(c)
  Constant18/1 -> tau_C/9(cf)
  Constant19/1 -> tau_C/10(CL_alpha)
  Constant11/1 -> tau_AS/5(rho_he)
  tau_C/1(tau_C) -> Scope4/1, V_dot out/6(tau_C)
  Constant15/1 -> MATLAB Function11/5(FVN)
  Constant12/1 -> MATLAB Function11/4(MVN)
  [delta_r] -> tau_C/5(delta_r)
  Constant21/1 -> tau_C/11(L_hull)
  [r] -> MATLAB Function11/2(r)
  In13/1 -> [fProp1]
  In14/1 -> [fProp2]
  In15/1 -> [Prop1_alpha]
  In16/1 -> [Prop2_alpha]
  In17/1 -> [delta_e]
  delta_r/1 -> [delta_r]
  [fProp2] -> MATLAB Function7/4(fProp2)
  [Prop1_alpha] -> MATLAB Function7/6(Prop1_alpha)
  [Prop2_alpha] -> MATLAB Function7/7(Prop2_alpha)
  [q] -> MATLAB Function11/3(q)
  MATLAB Function7/1(tau_Th) -> V_dot out/9(tau_Th)

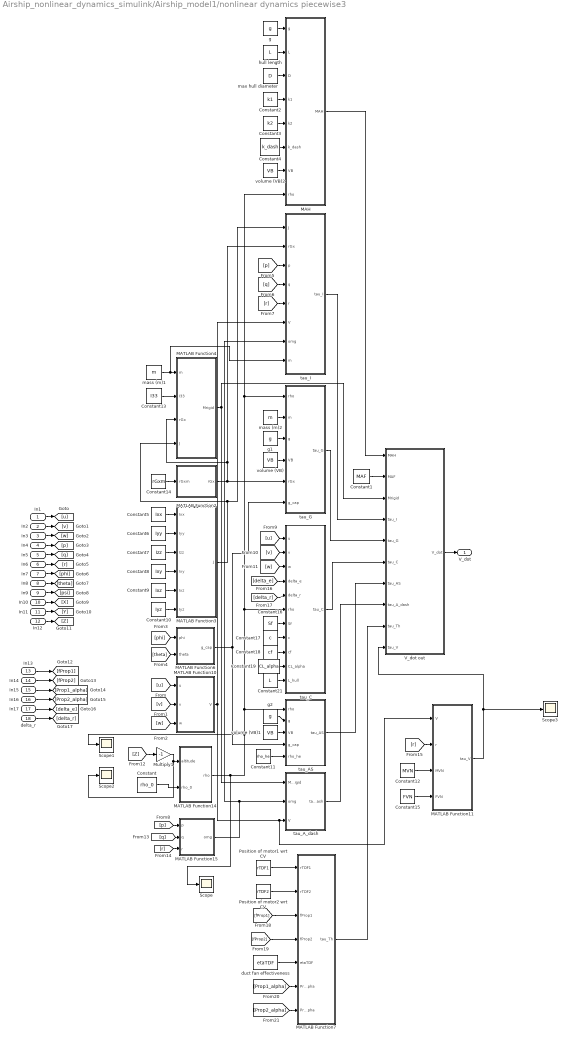
== system Airship_nonlinear_dynamics_simulink/Airship_model1/nonlinear dynamics piecewise3 ==
  In1 : Inport
  In2 : Inport  Port=2
  In3 : Inport  Port=3
  In4 : Inport  Port=4
  In5 : Inport  Port=5
  In6 : Inport  Port=6
  In7 : Inport  Port=7
  In8 : Inport  Port=8
  In9 : Inport  Port=9
  In10 : Inport  Port=10
  In11 : Inport  Port=11
  In12 : Inport  Port=12
  In13 : Inport  Port=13
  In14 : Inport  Port=14
  In15 : Inport  Port=15
  In16 : Inport  Port=16
  In17 : Inport  Port=17
  delta_r : Inport  Port=18
  Constant : Constant  Value=rho_0
  Constant1 : Constant  Value=MAF
  Constant10 : Constant  Value=Iyz
  Constant11 : Constant  Value=rho_he
  Constant12 : Constant  Value=MVN
  Constant13 : Constant  Value=I33
  Constant14 : Constant  Value=rGxm
  Constant15 : Constant  Value=FVN
  Constant16 : Constant  Value=Sf
  Constant17 : Constant  Value=c
  Constant18 : Constant  Value=cf
  Constant19 : Constant  Value=CL_alpha
  Constant2 : Constant  Value=k1
  Constant21 : Constant  Value=L
  Constant3 : Constant  Value=k2
  Constant4 : Constant  Value=k_dash
  Constant5 : Constant  Value=Ixx
  Constant6 : Constant  Value=Iyy
  Constant7 : Constant  Value=Izz
  Constant8 : Constant  Value=Ixy
  Constant9 : Constant  Value=Ixz
  MAH : MATLAB Function  TreatAsAtomicUnit=on
  MATLAB Function10 : MATLAB Function  TreatAsAtomicUnit=on
  MATLAB Function11 : MATLAB Function  TreatAsAtomicUnit=on
  MATLAB Function14 : MATLAB Function  TreatAsAtomicUnit=on
  MATLAB Function15 : MATLAB Function  TreatAsAtomicUnit=on
  MATLAB Function2 : MATLAB Function  TreatAsAtomicUnit=on
  MATLAB Function3 : MATLAB Function  TreatAsAtomicUnit=on
  MATLAB Function4 : MATLAB Function  TreatAsAtomicUnit=on
  MATLAB Function6 : MATLAB Function  TreatAsAtomicUnit=on
  MATLAB Function7 : MATLAB Function  TreatAsAtomicUnit=on
  Multiply1 : Gain  Gain=-1
  Position of motor1 wrt CV : Constant  Value=rTDF1
  Position of motor2 wrt CV : Constant  Value=rTDF2
  Scope{,1..3} (4 alike) : Scope
  V_dot out : MATLAB Function  TreatAsAtomicUnit=on
  duct fan effectiveness : Constant  Value=etaTDF
  g : Constant  Value=g
  g1 : Constant  Value=g
  g2 : Constant  Value=g
  hull length : Constant  Value=L
  mass (m)1 : Constant  Value=m
  mass (m)2 : Constant  Value=m
  max hull diameter : Constant  Value=D
  tau_AS : MATLAB Function  TreatAsAtomicUnit=on
  tau_A_dash : MATLAB Function  TreatAsAtomicUnit=on
  tau_C : MATLAB Function  TreatAsAtomicUnit=on
  tau_G : MATLAB Function  TreatAsAtomicUnit=on
  tau_I : MATLAB Function  TreatAsAtomicUnit=on
  volume (VB) : Constant  Value=VB
  volume (VB)1 : Constant  Value=VB
  volume (VB)2 : Constant  Value=VB
  V_dot : Outport
  wires:
  V_dot out/1(V_dot) -> V_dot/1
  Constant1/1 -> V_dot out/2(MAF)
  In1/1 -> [u]
  In2/1 -> [v]
  In3/1 -> [w]
  In4/1 -> [p]
  In5/1 -> [q]
  In6/1 -> [r]
  In7/1 -> [phi]
  In8/1 -> [theta]
  In9/1 -> [psi]
  In10/1 -> [X]
  In11/1 -> [Y]
  In12/1 -> [Z]
  mass (m)1/1 -> tau_I/8(m), MATLAB Function4/1(m)
  mass (m)2/1 -> tau_G/2(m)
  Constant13/1 -> MATLAB Function4/2(I33)
  Constant14/1 -> MATLAB Function2/1(rGxm)
  MATLAB Function2/1(rGx) -> tau_G/5(rGx), MATLAB Function4/3(rGx), tau_I/2(rGx)
  MATLAB Function3/1(J) -> MATLAB Function4/4(J), tau_I/1(J)
  Constant6/1 -> MATLAB Function3/2(Iyy)
  Constant5/1 -> MATLAB Function3/1(Ixx)
  Constant7/1 -> MATLAB Function3/3(Izz)
  Constant8/1 -> MATLAB Function3/4(Ixy)
  Constant9/1 -> MATLAB Function3/5(Ixz)
  Constant10/1 -> MATLAB Function3/6(Iyz)
  [u] -> MATLAB Function10/1(u)
  [v] -> MATLAB Function10/2(v)
  [w] -> MATLAB Function10/3(w)
  [phi] -> MATLAB Function6/1(phi)
  [theta] -> MATLAB Function6/2(theta)
  g/1 -> MAH/1(g)
  hull length/1 -> MAH/2(L)
  max hull diameter/1 -> MAH/3(D)
  Constant2/1 -> MAH/4(k1)
  Constant3/1 -> MAH/5(k2)
  [p] -> tau_I/3(p)
  [q] -> tau_I/4(q)
  [r] -> tau_I/5(r)
  MATLAB Function14/1(rho) -> Scope1/1, MAH/8(rho), tau_G/1(rho), tau_C/6(rho), tau_AS/1(rho), Scope/1
  g1/1 -> tau_G/3(g)
  volume (VB)/1 -> tau_G/4(VB)
  MATLAB Function6/1(g_cap) -> tau_AS/4(g_cap), tau_G/6(g_cap)
  [u] -> tau_C/1(u)
  [v] -> tau_C/2(v)
  [w] -> tau_C/3(w)
  [delta_e] -> tau_C/4(delta_e)
  [Z] -> Multiply1/1
  Multiply1/1 -> Scope2/1, MATLAB Function14/1(altitude)
  g2/1 -> tau_AS/2(g)
  volume (VB)1/1 -> tau_AS/3(VB)
  MATLAB Function4/1(Mrigid) -> tau_A_dash/1(MA_rigid), V_dot out/3(Mrigid)
  [p] -> MATLAB Function15/1(p)
  [q] -> MATLAB Function15/2(q)
  [r] -> MATLAB Function15/3(r)
  MATLAB Function15/1(omg) -> tau_I/7(omg), tau_A_dash/2(omg)
  Position of motor1 wrt CV/1 -> MATLAB Function7/1(rTDF1)
  Position of motor2 wrt CV/1 -> MATLAB Function7/2(rTDF2)
  duct fan effectiveness/1 -> MATLAB Function7/5(etaTDF)
  [fProp1] -> MATLAB Function7/3(fProp1)
  MATLAB Function10/1(V) -> MATLAB Function11/1(V), tau_A_dash/3(V), tau_I/6(V)
  Constant4/1 -> MAH/6(k_dash)
  MAH/1(MAH) -> V_dot out/1(MAH)
  tau_I/1(tau_I) -> V_dot out/4(tau_I)
  tau_G/1(tau_G) -> V_dot out/5(tau_G)
  tau_AS/1(tau_AS) -> V_dot out/7(tau_AS)
  tau_A_dash/1(tau_A_dash) -> V_dot out/8(tau_A_dash)
  MATLAB Function7/1(tau_Th) -> V_dot out/9(tau_Th)
  MATLAB Function11/1(tau_V) -> Scope3/1, V_dot out/10(tau_V)
  volume (VB)2/1 -> MAH/7(VB)
  Constant/1 -> MATLAB Function14/2(rho_0)
  Constant16/1 -> tau_C/7(Sf)
  Constant17/1 -> tau_C/8(c)
  Constant18/1 -> tau_C/9(cf)
  Constant19/1 -> tau_C/10(CL_alpha)
  Constant11/1 -> tau_AS/5(rho_he)
  tau_C/1(tau_C) -> V_dot out/6(tau_C)
  Constant15/1 -> MATLAB Function11/4(FVN)
  Constant12/1 -> MATLAB Function11/3(MVN)
  [delta_r] -> tau_C/5(delta_r)
  Constant21/1 -> tau_C/11(L_hull)
  [r] -> MATLAB Function11/2(r)
  In13/1 -> [fProp1]
  In14/1 -> [fProp2]
  In15/1 -> [Prop1_alpha]
  In16/1 -> [Prop2_alpha]
  In17/1 -> [delta_e]
  delta_r/1 -> [delta_r]
  [fProp2] -> MATLAB Function7/4(fProp2)
  [Prop1_alpha] -> MATLAB Function7/6(Prop1_alpha)
  [Prop2_alpha] -> MATLAB Function7/7(Prop2_alpha)

== matlab function Airship_nonlinear_dynamics_simulink/Position wrt earth1 ==
  data: u input; XYZ_dot output; v input; w input; phi input; theta input; psi input
function XYZ_dot = position_wrt_Earth(u,v,w,phi,theta,psi)


R_be = [cos(theta)*cos(psi) , sin(theta)*sin(phi)*cos(psi) - cos(theta)*sin(psi), cos(phi)*cos(psi)*sin(theta)+ sin(phi)*sin(psi); ...
    cos(theta)*sin(psi), sin(phi)*sin(theta)*sin(psi) + cos(phi)*cos(psi), cos(phi)*sin(theta)*sin(psi) - sin(phi)*cos(psi); ...
    -sin(theta) , sin(phi)*cos(theta) , cos(phi)*cos(theta)];

body_velocity = [u; v; w];
XYZ_dot = transpose(R_be*body_velocity);
end

== matlab function Airship_nonlinear_dynamics_simulink/nonlinear dynamics piecewise/tau_G ==
  data: rho input; tau_G output size=[6, 1]; m input; g input; VB input; rGx input; g_cap input
function tau_G = fcn(rho, m, g, VB, rGx, g_cap)
%% Gravitational forces and moments


w = m*g;
B = VB*rho*g;
FG = w*g_cap; % Weight component in body frame (N)
tau_G = [FG; rGx*FG];

== matlab function Airship_nonlinear_dynamics_simulink/nonlinear dynamics piecewise/MATLAB Function2 ==
  data: rGxm input; rGx output
function rGx = fcn(rGxm)
rGx = [0 -rGxm(3) rGxm(2) ; rGxm(3) 0 -rGxm(1) ; -rGxm(2) rGxm(1) 0];

== matlab function Airship_nonlinear_dynamics_simulink/nonlinear dynamics piecewise/MATLAB Function3 ==
  data: Ixx input; J output; Iyy input; Izz input; Ixy input; Ixz input; Iyz input
function J = fcn(Ixx, Iyy, Izz, Ixy, Ixz, Iyz)
J = [ Ixx, Ixy, Ixz ; Ixy, Iyy, Iyz ; Ixz, Iyz, Izz];

== matlab function Airship_nonlinear_dynamics_simulink/nonlinear dynamics piecewise/MATLAB Function4 ==
  data: m input; Mrigid output; I33 input; rGx input; J input
function Mrigid = fcn(m, I33, rGx, J)
Mrigid = [m*I33, -m*rGx; m*rGx,  J];

== matlab function Airship_nonlinear_dynamics_simulink/nonlinear dynamics piecewise/tau_AS ==
  data: rho input; tau_AS output size=[6, 1]; g input; VB input; g_cap input
function tau_AS = fcn(rho, g, VB, g_cap)
%% Aerostatic forces and moments

% first three are forces along x y z
% next three are moments along x y z 
rv = [0 0 0]'; %Since body frame is established at CV, the position ...
FAS = -rho*g*VB*g_cap; %Aerostatic forces N
tau_AS = [FAS; cross(rv,FAS)]; %Aerostatic forces and moments

== matlab function Airship_nonlinear_dynamics_simulink/nonlinear dynamics piecewise/MATLAB Function6 ==
  data: phi input; g_cap output; theta input
function g_cap = fcn(phi, theta)
g_cap = [-sin(theta), cos(theta)*sin(phi), cos(theta)*cos(phi)]';

== matlab function Airship_nonlinear_dynamics_simulink/nonlinear dynamics piecewise/MATLAB Function7 ==
  data: rTDF1 input; tau_Th output; rTDF2 input; fTDF input; etaTDF input; rTTP input; fTTP input; etaTP input
function tau_Th = fcn(rTDF1, rTDF2, fTDF, etaTDF, rTTP,  fTTP,  etaTP)
%% Airship thrust force and moments


FTDF1 = etaTDF * [fTDF 0 0 ]'; %Thrust force N
FTDF2 = etaTDF * [fTDF 0 0 ]';
FTDF = FTDF1+FTDF2;
MTDF1 = cross(rTDF1, FTDF1); %Moments N-m
MTDF2 = cross(rTDF2, FTDF2);
MTDF = MTDF1 + MTDF2;


FTTP = etaTP* [fTTP 0 0 ]';
MTTP = cross(rTTP, FTTP);

FT = FTTP + FTDF;
MT = MTTP + MTDF;
tau_Th = [FT; MT];

== matlab function Airship_nonlinear_dynamics_simulink/nonlinear dynamics piecewise/MAH ==
  data: MAH output; g input; L input; D input; k1 input; k2 input; k_dash input; VB input; rho input
function MAH = fcn(g, L, D, k1, k2, k_dash, VB, rho)
%% Estimation of added mass matrix
% MAH - added mass of airship hull
B = VB*rho*g; %Bouyancy force
m_dash = B/g;
%I_dash = sum(m_dash * (L.^2 + D^2) / 20); 
I_dash = (m_dash * (L.^2 + D^2) / 20); 

mH11 = k1*m_dash;
mH22 = k2*m_dash;
mH33 = mH22;
mH44 = 0;
mH55 = k_dash*I_dash;
mH66 = mH55;
mH = [mH11, mH22, mH33, mH44, mH55, mH66];

MAH = diag(mH); %6x6 diagonal matrix

== matlab function Airship_nonlinear_dynamics_simulink/nonlinear dynamics piecewise/tau_A_dash ==
  data: MA_rigid input; tau_A_dash output size=[6, 1]; omg input; V input
function tau_A_dash = fcn(MA_rigid, omg, V)
%% Aerodynamic forces and moments
% symmetric added mass axis
% Aerodynamic forces N and moments N-m

%extract components from the syymetric added mass axis
M11 = MA_rigid(1:3, 1:3);
M12 = MA_rigid(1:3, 4:6);
M21 = MA_rigid(4:6, 1:3);
M22 = MA_rigid(4:6, 4:6);

% Calc aero forces and moments

forces_due_to_rotation = cross(omg, (M11 * V + M12 *omg));
moments_due_to_translation = cross(V, (M11*V+M12*omg));
moments_due_to_rotation = cross (omg, (M21*V + M22*omg));

tau_A_dash = zeros(6,1);
%combine into aero forces and moments (sign change - to +)
tau_A_dash = [forces_due_to_rotation; moments_due_to_translation+moments_due_to_rotation];

== matlab function Airship_nonlinear_dynamics_simulink/nonlinear dynamics piecewise/MATLAB Function10 ==
  data: u input; V output; v input; w input
function V = fcn(u, v, w)
V = [u v w]';

== matlab function Airship_nonlinear_dynamics_simulink/nonlinear dynamics piecewise/MATLAB Function11 ==
  data: v input; tau_V output; w input
function tau_V = fcn(v, w)
%% Viscous forces
FVN = 0; %Viscous force
MVN = 0; %Viscous Moment
FV = FVN*[0 (-v/sqrt(v^2 + w^2)) (-w/sqrt(v^2 +w^2)) ]';
MV = MVN*[0 (w/sqrt(v^2 + w^2)) (-v/sqrt(v^2 +w^2)) ]';
tau_V = [FV; MV];

%tau_V = [0 0 0 0 0 0]'; %if slow speed

== matlab function Airship_nonlinear_dynamics_simulink/nonlinear dynamics piecewise/V_dot out ==
  data: MAH input; V_dot output; MAF input; tau_I input; tau_G input; tau_C input; tau_AS input; tau_A_dash input; tau_Th input; tau_V input
function V_dot = fcn(MAH, MAF, tau_I, tau_G, tau_C, tau_AS, tau_A_dash, tau_Th, tau_V)
%% Return
V_dot = zeros(6,1);
MA_rigid = (MAH+MAF);


%                                       +tau_Imp for gusts
V_dot = (MA_rigid + Mrigid) \ (tau_I + tau_G + tau_C + tau_AS + tau_A_dash + tau_Th + tau_V);

== matlab function Airship_nonlinear_dynamics_simulink/nonlinear dynamics piecewise/tau_C ==
  data: u input; tau_C output size=[6, 1]; v input; w input; delta input
function tau_C = fcn(u, v, w, delta)
%% Control forces and moments
% Constants

 V_bar  = sqrt(v^2 + u^2 + w^2) ; %true airspeed in m/s
 Sf = 65; % Surface area of the fin m^2
 c= 7 ; % Chord length of the fin
 cf = 3; %Flap chord
 
 S_FE = 65; %reference surface area m^2
 %
 delta = deg2rad(10);
 %lift curve slope
 CL_alpha = 5.7; %Change as needed
 
 %theoretical effectiveness factor tau
 theta_f = acos(2*cf/c -1);
 tau = 1- (theta_f - sin(theta_f)) /pi;
 
 %correction factor eta_d
 eta_d = 0.8; %simplified fucntion
 %3D effectiveness value
 k3D = 1.2; %example value
 %calc DeltaCL
 
 DeltaCL = CL_alpha *tau * eta_d * k3D * delta;
 
 DeltaCD = 1.7* (cf/c)^1.38 * (Sf / S_FE) * sin(delta)^2;
 
 %Moment calcs for each fin
 numerator = -2*sin(theta_f) - sin(2*theta_f);
 denominator = 8 * (pi - theta_f + sin(theta_f));
 
 ratio = numerator/denominator;
 
 DeltaCM1_4 = ratio*DeltaCL;
 
 %Deflection anges degrees
 theta = [45, 135, 225, 315];
 
 %initialize force and moment arrays
 
 Fx = zeros(1,4);
 Fy = zeros(1,4);
 Fz = zeros(1,4);
 
 L = zeros(1,4);
 M = zeros(1,4);
 N = zeros(1,4);
 
 %calc forces and moements for each fin
 
 for i = 1:4
     %conv theta to radians
     theta_rad = deg2rad(theta(i));
 
     %calc forces
     Fx(i) = -0.5 * rho * V_bar^2 *Sf*DeltaCD;
     Fy(i) = 0.5*rho*V_bar^2*Sf*(DeltaCL *sin(theta_rad)+ DeltaCD * cos(theta_rad));
     Fz(i) = -0.5 * rho * V_bar^2 *Sf*(DeltaCL *cos(theta_rad)- DeltaCD * sin(theta_rad));
 
     L(i) = Fz(i); %Assume y_i = 1 for simplicity
     M(i) = 0.5*rho*V_bar^2*Sf*c*DeltaCM1_4;
     N(i) = Fy(i); %Assume x_i = 1 for simplicity 
 end
 % Totals
 TotalFx = sum(Fx(:));
 TotalFy = sum(Fy(:));
 TotalFz = sum(Fz(:));
 
 TotalL = sum(L(:));
 TotalM = sum(M(:));
 TotalN = sum(N(:));

 tau_C = [TotalFx TotalFy TotalFz TotalL TotalM TotalN]';

%For natural response 
tau_C = [0 0 0 0 0 0]';

== matlab function Airship_nonlinear_dynamics_simulink/nonlinear dynamics piecewise/MATLAB Function14 ==
  data: altitude input; rho output
function rho = fcn(altitude)
%Atmosphere model
rho_0 = 1.225; %Density at sea level in kg/m3
H = 8400; %Scale height in meters;

%alitude range
%altitude = -airship(12); %linspace(0,12000, 500); %Altitude from 0 to 12000 m

density = rho_0 *exp(-altitude / H );
rho = density;

== matlab function Airship_nonlinear_dynamics_simulink/nonlinear dynamics piecewise/MATLAB Function15 ==
  data: p input; omg output; q input; r input
function omg = fcn(p, q, r)
omg = [p q r]';

== matlab function Airship_nonlinear_dynamics_simulink/Euler angle estimation3 ==
  data: phi input; EA_dot output; theta input; psi input; p input; q input; r input
function EA_dot = Euler_angle_estimation(phi, theta, psi,p, q, r)


E_dot = [1, sin(phi)* tan(theta) , cos(phi)*tan(theta);
         0, cos(phi) , -sin(phi);
         0, sin(phi)/cos(theta), cos(phi)/cos(theta)];

body_rates = [p; q; r];

EA_dot = transpose(E_dot*body_rates);

end

== matlab function Airship_nonlinear_dynamics_simulink/Position wrt earth3 ==
  data: u input; XYZ_dot output; v input; w input; phi input; theta input; psi input
function XYZ_dot = position_wrt_Earth(u,v,w,phi,theta,psi)


R_be = [cos(theta)*cos(psi) , sin(theta)*sin(phi)*cos(psi) - cos(theta)*sin(psi), cos(phi)*cos(psi)*sin(theta)+ sin(phi)*sin(psi); ...
    cos(theta)*sin(psi), sin(phi)*sin(theta)*sin(psi) + cos(phi)*cos(psi), cos(phi)*sin(theta)*sin(psi) - sin(phi)*cos(psi); ...
    -sin(theta) , sin(phi)*cos(theta) , cos(phi)*cos(theta)];

body_velocity = [u; v; w];
XYZ_dot = transpose(R_be*body_velocity);
end

== matlab function Airship_nonlinear_dynamics_simulink/nonlinear dynamics piecewise1/MAH ==
  data: MAH output; g input; L input; D input; k1 input; k2 input; k_dash input; VB input; rho input
function MAH = fcn(g, L, D, k1, k2, k_dash, VB, rho)
%% Estimation of added mass matrix
% MAH - added mass of airship hull
B = VB*rho*g; %Bouyancy force
m_dash = B/g;
%I_dash = sum(m_dash * (L.^2 + D^2) / 20); 
I_dash = (m_dash * (L.^2 + D^2) / 20); 

mH11 = k1*m_dash;
mH22 = k2*m_dash;
mH33 = mH22;
mH44 = 0;
mH55 = k_dash*I_dash;
mH66 = mH55;
mH = [mH11, mH22, mH33, mH44, mH55, mH66];

MAH = diag(mH); %6x6 diagonal matrix
end

== matlab function Airship_nonlinear_dynamics_simulink/nonlinear dynamics piecewise1/MATLAB Function10 ==
  data: u input; V output; v input; w input
function V = fcn(u, v, w)
V = [u v w]';
end

== matlab function Airship_nonlinear_dynamics_simulink/nonlinear dynamics piecewise1/MATLAB Function11 ==
  data: V input; r input; tau_V output size=[6,1]; MVN input; FVN input
 function tau_V = fcn(V, r, MVN, FVN)
 u= V(1); 
 v = V(2);
 w= V(3);

 if v == 0 && w == 0
     FV = [0 0 0]';
     MV = [0 0 0]';
 else
     FV = FVN.*[-u (-v) (-w) ]';
     %FV = FVN*[0 (-v/sqrt(v^2 + w^2)) (-w/sqrt(v^2 +w^2)) ]';
     %MV = MVN*[0 (w/sqrt(v^2 + w^2)) (-v/sqrt(v^2 +w^2)) ]';
    MV = MVN.*[0 (w) (-v) ]'; %make first element function of p if roll oscilations persists

 end
 MV(3) = MV(3) - MVN(3) * r; 
 tau_V = [FV; MV];
 %tau_V = [0 0 0 0 0 0]'; %if slow speed
 
 end

== matlab function Airship_nonlinear_dynamics_simulink/nonlinear dynamics piecewise1/MATLAB Function14 ==
  data: altitude input; rho output; rho_0 input
function rho = fcn(altitude, rho_0)
    % Constants
    T0 = 288.15;     % K
    L = 0.0065;      % K/m
    g = 9.80665;     % m/s^2
    R = 287.05;      % J/kg.K
%altitude = max(0, altitude);  % keep ≥ 0, but not forcefully clipped
    term = 1 - (L * altitude) / T0;
%rho= rho_0;
    if term <= 0
        rho = 0;
    else
       rho = rho_0 * term^(g / (R * L));
    end
end

== matlab function Airship_nonlinear_dynamics_simulink/nonlinear dynamics piecewise1/MATLAB Function15 ==
  data: p input; omg output; q input; r input
function omg = fcn(p, q, r)
omg = [p q r]';
end

== matlab function Airship_nonlinear_dynamics_simulink/nonlinear dynamics piecewise1/MATLAB Function2 ==
  data: rGxm input; rGx output
function rGx = fcn(rGxm)
rGx = [0 -rGxm(3) rGxm(2) ; rGxm(3) 0 -rGxm(1) ; -rGxm(2) rGxm(1) 0];

end

== matlab function Airship_nonlinear_dynamics_simulink/nonlinear dynamics piecewise1/MATLAB Function3 ==
  data: Ixx input; J output; Iyy input; Izz input; Ixy input; Ixz input; Iyz input
function J = fcn(Ixx, Iyy, Izz, Ixy, Ixz, Iyz)
J = [ Ixx, Ixy, Ixz ; Ixy, Iyy, Iyz ; Ixz, Iyz, Izz];
end

== matlab function Airship_nonlinear_dynamics_simulink/nonlinear dynamics piecewise1/MATLAB Function4 ==
  data: m input; Mrigid output; I33 input; rGx input; J input
function Mrigid = fcn(m, I33, rGx, J)
Mrigid = [m*I33, -m*rGx; m*rGx,  J];

end
